simulink library "halout"  (R2021b)
settings: Solver=VariableStepAuto  StartTime=0.0  StopTime=10.0  RelTol=1e-3
undefined symbols (not defined in the file): C_TASK_5MS_S, FALSE, KHAL_CAN1FD1APS3E2E_flg, KHAL_CAN1FD1APS3TxReq_flg, KHAL_CAN1FD1VCU2E2E_flg, KHAL_CAN1FD1VCU2TxReq_flg, KHAL_CAN1FD1VCU3E2E_flg, KHAL_CAN1FD1VCU3TxReq_flg, KHAL_CAN1TxReq_flg, KHAL_CAN1VMCFCM1E2E_flg, KHAL_CAN1VMCFCM1TxReq_flg, KHAL_CAN2TxReq_flg, KHAL_CAN3FD3VCU1toNIDECTxReq_flg, KHAL_CAN3FD3VCU1TxReq_flg, KHAL_CAN3FD3VCU2E2E_flg, KHAL_CAN3FD3VCU2toNIDECE2E_flg, KHAL_CAN3FD3VCU2toNIDECTxReq_flg, KHAL_CAN3FD3VCU2TxReq_flg, KHAL_CAN3TxReq_flg, KHAL_CAN4FD4CE1000E2E_flg, KHAL_CAN4FD4CE1000TxReq_flg, KHAL_CAN4TxReq_flg, KHAL_CAN5TxReq_flg, KHAL_CAN6FD6APS3E2E_flg, KHAL_CAN6FD6APS3TxReq_flg, KHAL_CAN6FD6VCU2E2E_flg, KHAL_CAN6FD6VCU2TxReq_flg, KHAL_CAN6TxReq_flg, ONE_INT, TRUE, ZERO_INT
libraries: FVT_lib x551, simulink x244
(part 22 of 26)

== system halout/HAL_OUT/CAN4/FD4_CE100_0_0x116/Byte_26 ==
  APS_Sta_System : Inport
  CTDLockSW : Inport  Port=2
  CTDUnlockSW : Inport  Port=3
  FDC_VMC_VehPitchAngle_Sta : Inport  Port=4
  BitwiseOR : simulink/Logic and Bit Operations/Bitwise Operator  logicop=OR  UseBitMask=off  NumInputPorts=4  BitMask=bin2dec('11011001')  BitMaskRealWorld=Stored Integer
  SignalPack : FVT_lib/hal/SignalPack  RightShiftCnt=0  BitMask=2^3-1  LeftShiftCnt=3
  SignalPack1 : FVT_lib/hal/SignalPack  RightShiftCnt=0  BitMask=2^1-1  LeftShiftCnt=7
  SignalPack2 : FVT_lib/hal/SignalPack  RightShiftCnt=0  BitMask=2^1-1  LeftShiftCnt=6
  SignalPack3 : FVT_lib/hal/SignalPack  RightShiftCnt=0  BitMask=2^3-1  LeftShiftCnt=0
  UnitConverter{,1..7} (8 alike) : DataTypeConversion  OutDataTypeStr=uint8  RndMeth=Round
  Byte_26 : Outport
  wires:
  BitwiseOR/1 -> Byte_26/1
  UnitConverter/1 -> BitwiseOR/1
  SignalPack/1 -> UnitConverter/1
  UnitConverter1/1 -> SignalPack/1
  APS_Sta_System/1 -> UnitConverter1/1
  UnitConverter2/1 -> BitwiseOR/2
  SignalPack1/1 -> UnitConverter2/1
  UnitConverter3/1 -> SignalPack1/1
  CTDLockSW/1 -> UnitConverter3/1
  UnitConverter4/1 -> BitwiseOR/3
  SignalPack2/1 -> UnitConverter4/1
  UnitConverter5/1 -> SignalPack2/1
  CTDUnlockSW/1 -> UnitConverter5/1
  UnitConverter6/1 -> BitwiseOR/4
  SignalPack3/1 -> UnitConverter6/1
  UnitConverter7/1 -> SignalPack3/1
  FDC_VMC_VehPitchAngle_Sta/1 -> UnitConverter7/1

== system halout/HAL_OUT/CAN4/FD4_CE100_0_0x116/Byte_27 ==
  CtrlDrPwrStbA2 : Inport
  Tailgate_SW : Inport  Port=2
  BitwiseOR : simulink/Logic and Bit Operations/Bitwise Operator  logicop=OR  UseBitMask=off  NumInputPorts=2  BitMask=bin2dec('11011001')  BitMaskRealWorld=Stored Integer
  SignalPack : FVT_lib/hal/SignalPack  RightShiftCnt=0  BitMask=2^1-1  LeftShiftCnt=6
  SignalPack1 : FVT_lib/hal/SignalPack  RightShiftCnt=0  BitMask=2^1-1  LeftShiftCnt=7
  UnitConverter{,1..3} (4 alike) : DataTypeConversion  OutDataTypeStr=uint8  RndMeth=Round
  Byte_27 : Outport
  wires:
  BitwiseOR/1 -> Byte_27/1
  UnitConverter/1 -> BitwiseOR/1
  SignalPack/1 -> UnitConverter/1
  UnitConverter1/1 -> SignalPack/1
  CtrlDrPwrStbA2/1 -> UnitConverter1/1
  UnitConverter2/1 -> BitwiseOR/2
  SignalPack1/1 -> UnitConverter2/1
  UnitConverter3/1 -> SignalPack1/1
  Tailgate_SW/1 -> UnitConverter3/1

== system halout/HAL_OUT/CAN4/FD4_CE100_0_0x116/Byte_3 ==
  H_Beam_ADB : Inport
  PwrSta : Inport  Port=2
  ReBrakeLPReq : Inport  Port=3
  ShiftGearPosn : Inport  Port=4
  BitwiseOR : simulink/Logic and Bit Operations/Bitwise Operator  logicop=OR  UseBitMask=off  NumInputPorts=4  BitMask=bin2dec('11011001')  BitMaskRealWorld=Stored Integer
  SignalPack : FVT_lib/hal/SignalPack  RightShiftCnt=0  BitMask=2^1-1  LeftShiftCnt=0
  SignalPack1 : FVT_lib/hal/SignalPack  RightShiftCnt=0  BitMask=2^3-1  LeftShiftCnt=2
  SignalPack2 : FVT_lib/hal/SignalPack  RightShiftCnt=0  BitMask=2^1-1  LeftShiftCnt=1
  SignalPack3 : FVT_lib/hal/SignalPack  RightShiftCnt=0  BitMask=2^3-1  LeftShiftCnt=5
  UnitConverter{,1..7} (8 alike) : DataTypeConversion  OutDataTypeStr=uint8  RndMeth=Round
  Byte_3 : Outport
  wires:
  BitwiseOR/1 -> Byte_3/1
  UnitConverter/1 -> BitwiseOR/1
  SignalPack/1 -> UnitConverter/1
  UnitConverter1/1 -> SignalPack/1
  H_Beam_ADB/1 -> UnitConverter1/1
  UnitConverter2/1 -> BitwiseOR/2
  SignalPack1/1 -> UnitConverter2/1
  UnitConverter3/1 -> SignalPack1/1
  PwrSta/1 -> UnitConverter3/1
  UnitConverter4/1 -> BitwiseOR/3
  SignalPack2/1 -> UnitConverter4/1
  UnitConverter5/1 -> SignalPack2/1
  ReBrakeLPReq/1 -> UnitConverter5/1
  UnitConverter6/1 -> BitwiseOR/4
  SignalPack3/1 -> UnitConverter6/1
  UnitConverter7/1 -> SignalPack3/1
  ShiftGearPosn/1 -> UnitConverter7/1

== system halout/HAL_OUT/CAN4/FD4_CE100_0_0x116/Byte_4 ==
  DKCTimeSN : Inport
  BitwiseOR : simulink/Logic and Bit Operations/Bitwise Operator  logicop=OR  UseBitMask=off  BitMask=bin2dec('11011001')  BitMaskRealWorld=Stored Integer
  SignalPack : FVT_lib/hal/SignalPack  RightShiftCnt=24  BitMask=2^8-1  LeftShiftCnt=0
  UnitConverter : DataTypeConversion  OutDataTypeStr=uint8  RndMeth=Round
  UnitConverter1 : DataTypeConversion  OutDataTypeStr=uint32  RndMeth=Round
  Byte_4 : Outport
  wires:
  BitwiseOR/1 -> Byte_4/1
  UnitConverter/1 -> BitwiseOR/1
  SignalPack/1 -> UnitConverter/1
  UnitConverter1/1 -> SignalPack/1
  DKCTimeSN/1 -> UnitConverter1/1

== system halout/HAL_OUT/CAN4/FD4_CE100_0_0x116/Byte_5 ==
  DKCTimeSN : Inport
  BitwiseOR : simulink/Logic and Bit Operations/Bitwise Operator  logicop=OR  UseBitMask=off  BitMask=bin2dec('11011001')  BitMaskRealWorld=Stored Integer
  SignalPack : FVT_lib/hal/SignalPack  RightShiftCnt=16  BitMask=2^8-1  LeftShiftCnt=0
  UnitConverter : DataTypeConversion  OutDataTypeStr=uint8  RndMeth=Round
  UnitConverter1 : DataTypeConversion  OutDataTypeStr=uint32  RndMeth=Round
  Byte_5 : Outport
  wires:
  BitwiseOR/1 -> Byte_5/1
  UnitConverter/1 -> BitwiseOR/1
  SignalPack/1 -> UnitConverter/1
  UnitConverter1/1 -> SignalPack/1
  DKCTimeSN/1 -> UnitConverter1/1

== system halout/HAL_OUT/CAN4/FD4_CE100_0_0x116/Byte_6 ==
  DKCTimeSN : Inport
  BitwiseOR : simulink/Logic and Bit Operations/Bitwise Operator  logicop=OR  UseBitMask=off  BitMask=bin2dec('11011001')  BitMaskRealWorld=Stored Integer
  SignalPack : FVT_lib/hal/SignalPack  RightShiftCnt=8  BitMask=2^8-1  LeftShiftCnt=0
  UnitConverter : DataTypeConversion  OutDataTypeStr=uint8  RndMeth=Round
  UnitConverter1 : DataTypeConversion  OutDataTypeStr=uint32  RndMeth=Round
  Byte_6 : Outport
  wires:
  BitwiseOR/1 -> Byte_6/1
  UnitConverter/1 -> BitwiseOR/1
  SignalPack/1 -> UnitConverter/1
  UnitConverter1/1 -> SignalPack/1
  DKCTimeSN/1 -> UnitConverter1/1

== system halout/HAL_OUT/CAN4/FD4_CE100_0_0x116/Byte_7 ==
  DKCTimeSN : Inport
  BitwiseOR : simulink/Logic and Bit Operations/Bitwise Operator  logicop=OR  UseBitMask=off  BitMask=bin2dec('11011001')  BitMaskRealWorld=Stored Integer
  SignalPack : FVT_lib/hal/SignalPack  RightShiftCnt=0  BitMask=2^8-1  LeftShiftCnt=0
  UnitConverter : DataTypeConversion  OutDataTypeStr=uint8  RndMeth=Round
  UnitConverter1 : DataTypeConversion  OutDataTypeStr=uint32  RndMeth=Round
  Byte_7 : Outport
  wires:
  BitwiseOR/1 -> Byte_7/1
  UnitConverter/1 -> BitwiseOR/1
  SignalPack/1 -> UnitConverter/1
  UnitConverter1/1 -> SignalPack/1
  DKCTimeSN/1 -> UnitConverter1/1

== system halout/HAL_OUT/CAN4/FD4_CE100_0_0x116/Byte_8 ==
  TimeSNDKCFbk : Inport
  BitwiseOR : simulink/Logic and Bit Operations/Bitwise Operator  logicop=OR  UseBitMask=off  BitMask=bin2dec('11011001')  BitMaskRealWorld=Stored Integer
  SignalPack : FVT_lib/hal/SignalPack  RightShiftCnt=24  BitMask=2^8-1  LeftShiftCnt=0
  UnitConverter : DataTypeConversion  OutDataTypeStr=uint8  RndMeth=Round
  UnitConverter1 : DataTypeConversion  OutDataTypeStr=uint32  RndMeth=Round
  Byte_8 : Outport
  wires:
  BitwiseOR/1 -> Byte_8/1
  UnitConverter/1 -> BitwiseOR/1
  SignalPack/1 -> UnitConverter/1
  UnitConverter1/1 -> SignalPack/1
  TimeSNDKCFbk/1 -> UnitConverter1/1

== system halout/HAL_OUT/CAN4/FD4_CE100_0_0x116/Byte_9 ==
  TimeSNDKCFbk : Inport
  BitwiseOR : simulink/Logic and Bit Operations/Bitwise Operator  logicop=OR  UseBitMask=off  BitMask=bin2dec('11011001')  BitMaskRealWorld=Stored Integer
  SignalPack : FVT_lib/hal/SignalPack  RightShiftCnt=16  BitMask=2^8-1  LeftShiftCnt=0
  UnitConverter : DataTypeConversion  OutDataTypeStr=uint8  RndMeth=Round
  UnitConverter1 : DataTypeConversion  OutDataTypeStr=uint32  RndMeth=Round
  Byte_9 : Outport
  wires:
  BitwiseOR/1 -> Byte_9/1
  UnitConverter/1 -> BitwiseOR/1
  SignalPack/1 -> UnitConverter/1
  UnitConverter1/1 -> SignalPack/1
  TimeSNDKCFbk/1 -> UnitConverter1/1

== system halout/HAL_OUT/CAN4/FD4_CE100_0_0x116/CCCrlSta ==
  CCCrlSta : Inport
  Data Type Conversion : DataTypeConversion  OutDataTypeStr=uint8  RndMeth=Round
  CAN4_CC_Crl_Sta : Outport
  wires:
  Data Type Conversion/1 -> CAN4_CC_Crl_Sta/1
  CCCrlSta/1 -> Data Type Conversion/1

== system halout/HAL_OUT/CAN4/FD4_CE100_0_0x116/CRC8_IfAction_Tx ==
  CAN_E2E_flg : Inport
  DataID1 : Inport  Port=2
  DataID2 : Inport  Port=3
  RawData : Inport  Port=4
  Data Type Conversion : DataTypeConversion  OutDataTypeStr=uint8
  If : If
  If Action Subsystem : Subsystem  TreatAsAtomicUnit=on
  If Action Subsystem1 : Subsystem  TreatAsAtomicUnit=on
  Merge : Merge
  CRC8 : Outport
  wires:
  If/2 -> If Action Subsystem/Action
  If/1 -> If Action Subsystem1/Action
  CAN_E2E_flg/1 -> [CAN_E2E_flg]
  DataID1/1 -> [DataID1]
  DataID2/1 -> [DataID2]
  RawData/1 -> [RawData]
  [CAN_E2E_flg] -> Data Type Conversion/1
  [DataID1] -> If Action Subsystem1/1(CAN_E2E_ID1)
  [DataID2] -> If Action Subsystem1/2(CAN_E2E_ID2)
  [RawData] -> If Action Subsystem1/3(Byte1)
  [RawData] -> If Action Subsystem/1(Byte1)
  If Action Subsystem1/1(CRC8_E2EResult) -> Merge/1
  If Action Subsystem/1(CRC8_Result) -> Merge/2
  Merge/1 -> CRC8/1
  Data Type Conversion/1 -> If/1

== system halout/HAL_OUT/CAN4/FD4_CE100_0_0x116/CSVCU1CAN4 ==
  CSVCU1CAN4 : Inport
  Data Type Conversion : DataTypeConversion  OutDataTypeStr=uint8  RndMeth=Round
  CAN4_CS_VCU1_CAN4 : Outport
  wires:
  Data Type Conversion/1 -> CAN4_CS_VCU1_CAN4/1
  CSVCU1CAN4/1 -> Data Type Conversion/1

== system halout/HAL_OUT/CAN4/FD4_CE100_0_0x116/CTDCtrl ==
  CTDCtrl : Inport
  Data Type Conversion : DataTypeConversion  OutDataTypeStr=uint8  RndMeth=Round
  CAN4_CTDCtrl : Outport
  wires:
  Data Type Conversion/1 -> CAN4_CTDCtrl/1
  CTDCtrl/1 -> Data Type Conversion/1

== system halout/HAL_OUT/CAN4/FD4_CE100_0_0x116/CTDLockSW ==
  CTDLockSW : Inport
  Data Type Conversion : DataTypeConversion  OutDataTypeStr=uint8  RndMeth=Round
  CAN4_CTDLockSW : Outport
  wires:
  Data Type Conversion/1 -> CAN4_CTDLockSW/1
  CTDLockSW/1 -> Data Type Conversion/1

== system halout/HAL_OUT/CAN4/FD4_CE100_0_0x116/CTDUnlockSW ==
  CTDUnlockSW : Inport
  Data Type Conversion : DataTypeConversion  OutDataTypeStr=uint8  RndMeth=Round
  CAN4_CTDUnlockSW : Outport
  wires:
  Data Type Conversion/1 -> CAN4_CTDUnlockSW/1
  CTDUnlockSW/1 -> Data Type Conversion/1

== system halout/HAL_OUT/CAN4/FD4_CE100_0_0x116/CrashDetd ==
  CrashDetd : Inport
  Data Type Conversion : DataTypeConversion  OutDataTypeStr=uint8  RndMeth=Round
  CAN4_CrashDetd : Outport
  wires:
  Data Type Conversion/1 -> CAN4_CrashDetd/1
  CrashDetd/1 -> Data Type Conversion/1

== system halout/HAL_OUT/CAN4/FD4_CE100_0_0x116/CtrlDrPwrStbA2 ==
  CtrlDrPwrStbA2 : Inport
  Data Type Conversion : DataTypeConversion  OutDataTypeStr=uint8  RndMeth=Round
  CAN4_CtrlDrPwrStbA2 : Outport
  wires:
  Data Type Conversion/1 -> CAN4_CtrlDrPwrStbA2/1
  CtrlDrPwrStbA2/1 -> Data Type Conversion/1

== system halout/HAL_OUT/CAN4/FD4_CE100_0_0x116/CtrlFrBMSCCUCIR ==
  CtrlFrBMSCCUCIR : Inport
  Data Type Conversion : DataTypeConversion  OutDataTypeStr=uint8  RndMeth=Round
  CAN4_CtrlFrBMSCCUCIR : Outport
  wires:
  Data Type Conversion/1 -> CAN4_CtrlFrBMSCCUCIR/1
  CtrlFrBMSCCUCIR/1 -> Data Type Conversion/1

== system halout/HAL_OUT/CAN4/FD4_CE100_0_0x116/CtrlFrEDUINVERTER ==
  CtrlFrEDUINVERTER : Inport
  Data Type Conversion : DataTypeConversion  OutDataTypeStr=uint8  RndMeth=Round
  CAN4_CtrlFrEDUINVERTER : Outport
  wires:
  Data Type Conversion/1 -> CAN4_CtrlFrEDUINVERTER/1
  CtrlFrEDUINVERTER/1 -> Data Type Conversion/1

== system halout/HAL_OUT/CAN4/FD4_CE100_0_0x116/CtrlFrIRC1 ==
  CtrlFrIRC1 : Inport
  Data Type Conversion : DataTypeConversion  OutDataTypeStr=uint8  RndMeth=Round
  CAN4_CtrlFrIRC1 : Outport
  wires:
  Data Type Conversion/1 -> CAN4_CtrlFrIRC1/1
  CtrlFrIRC1/1 -> Data Type Conversion/1

== system halout/HAL_OUT/CAN4/FD4_CE100_0_0x116/CtrlFrPwrStbA1P ==
  CtrlFrPwrStbA1P : Inport
  Data Type Conversion : DataTypeConversion  OutDataTypeStr=uint8  RndMeth=Round
  CAN4_CtrlFrPwrStbA1P : Outport
  wires:
  Data Type Conversion/1 -> CAN4_CtrlFrPwrStbA1P/1
  CtrlFrPwrStbA1P/1 -> Data Type Conversion/1

== system halout/HAL_OUT/CAN4/FD4_CE100_0_0x116/DKCAuthSta ==
  DKCAuthSta : Inport
  Data Type Conversion : DataTypeConversion  OutDataTypeStr=uint8  RndMeth=Round
  CAN4_DKCAuthSta : Outport
  wires:
  Data Type Conversion/1 -> CAN4_DKCAuthSta/1
  DKCAuthSta/1 -> Data Type Conversion/1

== system halout/HAL_OUT/CAN4/FD4_CE100_0_0x116/DKCTimeSN ==
  DKCTimeSN : Inport
  Data Type Conversion : DataTypeConversion  OutDataTypeStr=uint32  RndMeth=Round
  CAN4_DKCTimeSN : Outport
  wires:
  Data Type Conversion/1 -> CAN4_DKCTimeSN/1
  DKCTimeSN/1 -> Data Type Conversion/1

== system halout/HAL_OUT/CAN4/FD4_CE100_0_0x116/Dimmer ==
  Dimmer : Inport
  Data Type Conversion : DataTypeConversion  OutDataTypeStr=uint8  RndMeth=Round
  CAN4_Dimmer : Outport
  wires:
  Data Type Conversion/1 -> CAN4_Dimmer/1
  Dimmer/1 -> Data Type Conversion/1

== system halout/HAL_OUT/CAN4/FD4_CE100_0_0x116/DimmerEN ==
  DimmerEN : Inport
  Data Type Conversion : DataTypeConversion  OutDataTypeStr=uint8  RndMeth=Round
  CAN4_DimmerEN : Outport
  wires:
  Data Type Conversion/1 -> CAN4_DimmerEN/1
  DimmerEN/1 -> Data Type Conversion/1

== system halout/HAL_OUT/CAN4/FD4_CE100_0_0x116/DoorLockIND ==
  DoorLockIND : Inport
  Data Type Conversion : DataTypeConversion  OutDataTypeStr=uint8  RndMeth=Round
  CAN4_DoorLockIND : Outport
  wires:
  Data Type Conversion/1 -> CAN4_DoorLockIND/1
  DoorLockIND/1 -> Data Type Conversion/1

== system halout/HAL_OUT/CAN4/FD4_CE100_0_0x116/DrDoorSW ==
  DrDoorSW : Inport
  Data Type Conversion : DataTypeConversion  OutDataTypeStr=uint8  RndMeth=Round
  CAN4_DrDoorSW : Outport
  wires:
  Data Type Conversion/1 -> CAN4_DrDoorSW/1
  DrDoorSW/1 -> Data Type Conversion/1

== system halout/HAL_OUT/CAN4/FD4_CE100_0_0x116/DrSeatSta ==
  DrSeatSta : Inport
  Data Type Conversion : DataTypeConversion  OutDataTypeStr=uint8  RndMeth=Round
  CAN4_Dr_SeatSta : Outport
  wires:
  Data Type Conversion/1 -> CAN4_Dr_SeatSta/1
  DrSeatSta/1 -> Data Type Conversion/1

== system halout/HAL_OUT/CAN4/FD4_CE100_0_0x116/EquivAccPedalSWSta ==
  EquivAccPedalSWSta : Inport
  Data Type Conversion : DataTypeConversion  OutDataTypeStr=uint8  RndMeth=Round
  CAN4_EquivAccPedalSWSta : Outport
  wires:
  Data Type Conversion/1 -> CAN4_EquivAccPedalSWSta/1
  EquivAccPedalSWSta/1 -> Data Type Conversion/1

== system halout/HAL_OUT/CAN4/FD4_CE100_0_0x116/FDCVMCVehPitchAngleSta ==
  FDCVMCVehPitchAngleSta : Inport
  Data Type Conversion : DataTypeConversion  OutDataTypeStr=uint8  RndMeth=Round
  CAN4_FDC_VMC_VehPitchAngle_Sta : Outport
  wires:
  Data Type Conversion/1 -> CAN4_FDC_VMC_VehPitchAngle_Sta/1
  FDCVMCVehPitchAngleSta/1 -> Data Type Conversion/1

== system halout/HAL_OUT/CAN4/FD4_CE100_0_0x116/FDDKCVehDataErr ==
  FDDKCVehDataErr : Inport
  Data Type Conversion : DataTypeConversion  OutDataTypeStr=uint8  RndMeth=Round
  CAN4_FD_DKC_VehData_Err : Outport
  wires:
  Data Type Conversion/1 -> CAN4_FD_DKC_VehData_Err/1
  FDDKCVehDataErr/1 -> Data Type Conversion/1

== system halout/HAL_OUT/CAN4/FD4_CE100_0_0x116/FDDKCVehDataSta ==
  FDDKCVehDataSta : Inport
  Data Type Conversion : DataTypeConversion  OutDataTypeStr=uint8  RndMeth=Round
  CAN4_FD_DKC_VehData_Sta : Outport
  wires:
  Data Type Conversion/1 -> CAN4_FD_DKC_VehData_Sta/1
  FDDKCVehDataSta/1 -> Data Type Conversion/1

== system halout/HAL_OUT/CAN4/FD4_CE100_0_0x116/FDTBOXDTCDataErr ==
  FDTBOXDTCDataErr : Inport
  Data Type Conversion : DataTypeConversion  OutDataTypeStr=uint8  RndMeth=Round
  CAN4_FD_TBOX_DTCData_Err : Outport
  wires:
  Data Type Conversion/1 -> CAN4_FD_TBOX_DTCData_Err/1
  FDTBOXDTCDataErr/1 -> Data Type Conversion/1

== system halout/HAL_OUT/CAN4/FD4_CE100_0_0x116/FDTBOXDTCDataSta ==
  FDTBOXDTCDataSta : Inport
  Data Type Conversion : DataTypeConversion  OutDataTypeStr=uint8  RndMeth=Round
  CAN4_FD_TBOX_DTCData_Sta : Outport
  wires:
  Data Type Conversion/1 -> CAN4_FD_TBOX_DTCData_Sta/1
  FDTBOXDTCDataSta/1 -> Data Type Conversion/1

== system halout/HAL_OUT/CAN4/FD4_CE100_0_0x116/FDTBOXVehDataErr ==
  FDTBOXVehDataErr : Inport
  Data Type Conversion : DataTypeConversion  OutDataTypeStr=uint8  RndMeth=Round
  CAN4_FD_TBOX_VehData_Err : Outport
  wires:
  Data Type Conversion/1 -> CAN4_FD_TBOX_VehData_Err/1
  FDTBOXVehDataErr/1 -> Data Type Conversion/1

== system halout/HAL_OUT/CAN4/FD4_CE100_0_0x116/FDTBOXVehDataSta ==
  FDTBOXVehDataSta : Inport
  Data Type Conversion : DataTypeConversion  OutDataTypeStr=uint8  RndMeth=Round
  CAN4_FD_TBOX_VehData_Sta : Outport
  wires:
  Data Type Conversion/1 -> CAN4_FD_TBOX_VehData_Sta/1
  FDTBOXVehDataSta/1 -> Data Type Conversion/1

== system halout/HAL_OUT/CAN4/FD4_CE100_0_0x116/FrChargingDoorCtrl ==
  FrChargingDoorCtrl : Inport
  Data Type Conversion : DataTypeConversion  OutDataTypeStr=uint8  RndMeth=Round
  CAN4_Fr_ChargingDoorCtrl : Outport
  wires:
  Data Type Conversion/1 -> CAN4_Fr_ChargingDoorCtrl/1
  FrChargingDoorCtrl/1 -> Data Type Conversion/1

== system halout/HAL_OUT/CAN4/FD4_CE100_0_0x116/FrFogLamp ==
  FrFogLamp : Inport
  Data Type Conversion : DataTypeConversion  OutDataTypeStr=uint8  RndMeth=Round
  CAN4_Fr_FogLamp : Outport
  wires:
  Data Type Conversion/1 -> CAN4_Fr_FogLamp/1
  FrFogLamp/1 -> Data Type Conversion/1

== system halout/HAL_OUT/CAN4/FD4_CE100_0_0x116/FrWiperH ==
  FrWiperH : Inport
  Data Type Conversion : DataTypeConversion  OutDataTypeStr=uint8  RndMeth=Round
  CAN4_Fr_Wiper_H : Outport
  wires:
  Data Type Conversion/1 -> CAN4_Fr_Wiper_H/1
  FrWiperH/1 -> Data Type Conversion/1

== system halout/HAL_OUT/CAN4/FD4_CE100_0_0x116/FrWiperL ==
  FrWiperL : Inport
  Data Type Conversion : DataTypeConversion  OutDataTypeStr=uint8  RndMeth=Round
  CAN4_Fr_Wiper_L : Outport
  wires:
  Data Type Conversion/1 -> CAN4_Fr_Wiper_L/1
  FrWiperL/1 -> Data Type Conversion/1

== system halout/HAL_OUT/CAN4/FD4_CE100_0_0x116/HBeam ==
  HBeam : Inport
  Data Type Conversion : DataTypeConversion  OutDataTypeStr=uint8  RndMeth=Round
  CAN4_H_Beam : Outport
  wires:
  Data Type Conversion/1 -> CAN4_H_Beam/1
  HBeam/1 -> Data Type Conversion/1

== system halout/HAL_OUT/CAN4/FD4_CE100_0_0x116/HBeamADB ==
  HBeamADB : Inport
  Data Type Conversion : DataTypeConversion  OutDataTypeStr=uint8  RndMeth=Round
  CAN4_H_Beam_ADB : Outport
  wires:
  Data Type Conversion/1 -> CAN4_H_Beam_ADB/1
  HBeamADB/1 -> Data Type Conversion/1

== system halout/HAL_OUT/CAN4/FD4_CE100_0_0x116/HWResetSta ==
  HWResetSta : Inport
  Data Type Conversion : DataTypeConversion  OutDataTypeStr=uint8  RndMeth=Round
  CAN4_HWResetSta : Outport
  wires:
  Data Type Conversion/1 -> CAN4_HWResetSta/1
  HWResetSta/1 -> Data Type Conversion/1

== system halout/HAL_OUT/CAN4/FD4_CE100_0_0x116/HazardSW ==
  HazardSW : Inport
  Data Type Conversion : DataTypeConversion  OutDataTypeStr=uint8  RndMeth=Round
  CAN4_HazardSW : Outport
  wires:
  Data Type Conversion/1 -> CAN4_HazardSW/1
  HazardSW/1 -> Data Type Conversion/1

== system halout/HAL_OUT/CAN4/FD4_CE100_0_0x116/HoodSW ==
  HoodSW : Inport
  Data Type Conversion : DataTypeConversion  OutDataTypeStr=uint8  RndMeth=Round
  CAN4_HoodSW : Outport
  wires:
  Data Type Conversion/1 -> CAN4_HoodSW/1
  HoodSW/1 -> Data Type Conversion/1

== system halout/HAL_OUT/CAN4/FD4_CE100_0_0x116/HornCtrl ==
  HornCtrl : Inport
  Data Type Conversion : DataTypeConversion  OutDataTypeStr=uint8  RndMeth=Round
  CAN4_HornCtrl : Outport
  wires:
  Data Type Conversion/1 -> CAN4_HornCtrl/1
  HornCtrl/1 -> Data Type Conversion/1

== system halout/HAL_OUT/CAN4/FD4_CE100_0_0x116/LAPMWdwEnable ==
  LAPMWdwEnable : Inport
  Data Type Conversion : DataTypeConversion  OutDataTypeStr=uint8  RndMeth=Round
  CAN4_L_APM_WdwEnable : Outport
  wires:
  Data Type Conversion/1 -> CAN4_L_APM_WdwEnable/1
  LAPMWdwEnable/1 -> Data Type Conversion/1

== system halout/HAL_OUT/CAN4/FD4_CE100_0_0x116/LBSD ==
  LBSD : Inport
  Data Type Conversion : DataTypeConversion  OutDataTypeStr=uint8  RndMeth=Round
  CAN4_LBSD : Outport
  wires:
  Data Type Conversion/1 -> CAN4_LBSD/1
  LBSD/1 -> Data Type Conversion/1

== system halout/HAL_OUT/CAN4/FD4_CE100_0_0x116/LBeam ==
  LBeam : Inport
  Data Type Conversion : DataTypeConversion  OutDataTypeStr=uint8  RndMeth=Round
  CAN4_L_Beam : Outport
  wires:
  Data Type Conversion/1 -> CAN4_L_Beam/1
  LBeam/1 -> Data Type Conversion/1

== system halout/HAL_OUT/CAN4/FD4_CE100_0_0x116/LDRL ==
  LDRL : Inport
  Data Type Conversion : DataTypeConversion  OutDataTypeStr=uint8  RndMeth=Round
  CAN4_LDRL : Outport
  wires:
  Data Type Conversion/1 -> CAN4_LDRL/1
  LDRL/1 -> Data Type Conversion/1

== system halout/HAL_OUT/CAN4/FD4_CE100_0_0x116/LTurnLP ==
  LTurnLP : Inport
  Data Type Conversion : DataTypeConversion  OutDataTypeStr=uint8  RndMeth=Round
  CAN4_LTurnLP : Outport
  wires:
  Data Type Conversion/1 -> CAN4_LTurnLP/1
  LTurnLP/1 -> Data Type Conversion/1

== system halout/HAL_OUT/CAN4/FD4_CE100_0_0x116/LampPwr ==
  LampPwr : Inport
  Data Type Conversion : DataTypeConversion  OutDataTypeStr=uint8  RndMeth=Round
  CAN4_LampPwr : Outport
  wires:
  Data Type Conversion/1 -> CAN4_LampPwr/1
  LampPwr/1 -> Data Type Conversion/1

== system halout/HAL_OUT/CAN4/FD4_CE100_0_0x116/LockSetting ==
  LockSetting : Inport
  Data Type Conversion : DataTypeConversion  OutDataTypeStr=uint8  RndMeth=Round
  CAN4_LockSetting : Outport
  wires:
  Data Type Conversion/1 -> CAN4_LockSetting/1
  LockSetting/1 -> Data Type Conversion/1

== system halout/HAL_OUT/CAN4/FD4_CE100_0_0x116/MSACrlSta ==
  MSACrlSta : Inport
  Data Type Conversion : DataTypeConversion  OutDataTypeStr=uint8  RndMeth=Round
  CAN4_MSA_Crl_Sta : Outport
  wires:
  Data Type Conversion/1 -> CAN4_MSA_Crl_Sta/1
  MSACrlSta/1 -> Data Type Conversion/1

== system halout/HAL_OUT/CAN4/FD4_CE100_0_0x116/MirrorCtrl ==
  MirrorCtrl : Inport
  Data Type Conversion : DataTypeConversion  OutDataTypeStr=uint8  RndMeth=Round
  CAN4_MirrorCtrl : Outport
  wires:
  Data Type Conversion/1 -> CAN4_MirrorCtrl/1
  MirrorCtrl/1 -> Data Type Conversion/1

== system halout/HAL_OUT/CAN4/FD4_CE100_0_0x116/MirrorDefog ==
  MirrorDefog : Inport
  Data Type Conversion : DataTypeConversion  OutDataTypeStr=uint8  RndMeth=Round
  CAN4_MirrorDefog : Outport
  wires:
  Data Type Conversion/1 -> CAN4_MirrorDefog/1
  MirrorDefog/1 -> Data Type Conversion/1

== system halout/HAL_OUT/CAN4/FD4_CE100_0_0x116/PosLamp ==
  PosLamp : Inport
  Data Type Conversion : DataTypeConversion  OutDataTypeStr=uint8  RndMeth=Round
  CAN4_PosLamp : Outport
  wires:
  Data Type Conversion/1 -> CAN4_PosLamp/1
  PosLamp/1 -> Data Type Conversion/1

== system halout/HAL_OUT/CAN4/FD4_CE100_0_0x116/PsDoorSW ==
  PsDoorSW : Inport
  Data Type Conversion : DataTypeConversion  OutDataTypeStr=uint8  RndMeth=Round
  CAN4_PsDoorSW : Outport
  wires:
  Data Type Conversion/1 -> CAN4_PsDoorSW/1
  PsDoorSW/1 -> Data Type Conversion/1

== system halout/HAL_OUT/CAN4/FD4_CE100_0_0x116/PwrSta ==
  PwrSta : Inport
  Data Type Conversion : DataTypeConversion  OutDataTypeStr=uint8  RndMeth=Round
  CAN4_PwrSta : Outport
  wires:
  Data Type Conversion/1 -> CAN4_PwrSta/1
  PwrSta/1 -> Data Type Conversion/1

== system halout/HAL_OUT/CAN4/FD4_CE100_0_0x116/RBSD ==
  RBSD : Inport
  Data Type Conversion : DataTypeConversion  OutDataTypeStr=uint8  RndMeth=Round
  CAN4_RBSD : Outport
  wires:
  Data Type Conversion/1 -> CAN4_RBSD/1
  RBSD/1 -> Data Type Conversion/1

== system halout/HAL_OUT/CAN4/FD4_CE100_0_0x116/RCVCU1CAN4 ==
  RCVCU1CAN4 : Inport
  Data Type Conversion : DataTypeConversion  OutDataTypeStr=uint8  RndMeth=Round
  CAN4_RC_VCU1_CAN4 : Outport
  wires:
  Data Type Conversion/1 -> CAN4_RC_VCU1_CAN4/1
  RCVCU1CAN4/1 -> Data Type Conversion/1

== system halout/HAL_OUT/CAN4/FD4_CE100_0_0x116/RDRL ==
  RDRL : Inport
  Data Type Conversion : DataTypeConversion  OutDataTypeStr=uint8  RndMeth=Round
  CAN4_RDRL : Outport
  wires:
  Data Type Conversion/1 -> CAN4_RDRL/1
  RDRL/1 -> Data Type Conversion/1

== system halout/HAL_OUT/CAN4/FD4_CE100_0_0x116/RLDoorSW ==
  RLDoorSW : Inport
  Data Type Conversion : DataTypeConversion  OutDataTypeStr=uint8  RndMeth=Round
  CAN4_RLDoorSW : Outport
  wires:
  Data Type Conversion/1 -> CAN4_RLDoorSW/1
  RLDoorSW/1 -> Data Type Conversion/1

== system halout/HAL_OUT/CAN4/FD4_CE100_0_0x116/RRDoorSW ==
  RRDoorSW : Inport
  Data Type Conversion : DataTypeConversion  OutDataTypeStr=uint8  RndMeth=Round
  CAN4_RRDoorSW : Outport
  wires:
  Data Type Conversion/1 -> CAN4_RRDoorSW/1
  RRDoorSW/1 -> Data Type Conversion/1

== system halout/HAL_OUT/CAN4/FD4_CE100_0_0x116/RTurnLP ==
  RTurnLP : Inport
  Data Type Conversion : DataTypeConversion  OutDataTypeStr=uint8  RndMeth=Round
  CAN4_RTurnLP : Outport
  wires:
  Data Type Conversion/1 -> CAN4_RTurnLP/1
  RTurnLP/1 -> Data Type Conversion/1

== system halout/HAL_OUT/CAN4/FD4_CE100_0_0x116/ReBrakeLPReq ==
  ReBrakeLPReq : Inport
  Data Type Conversion : DataTypeConversion  OutDataTypeStr=uint8  RndMeth=Round
  CAN4_ReBrakeLPReq : Outport
  wires:
  Data Type Conversion/1 -> CAN4_ReBrakeLPReq/1
  ReBrakeLPReq/1 -> Data Type Conversion/1

== system halout/HAL_OUT/CAN4/FD4_CE100_0_0x116/ReverseLamp ==
  ReverseLamp : Inport
  Data Type Conversion : DataTypeConversion  OutDataTypeStr=uint8  RndMeth=Round
  CAN4_ReverseLamp : Outport
  wires:
  Data Type Conversion/1 -> CAN4_ReverseLamp/1
  ReverseLamp/1 -> Data Type Conversion/1

== system halout/HAL_OUT/CAN4/FD4_CE100_0_0x116/RoomLampH ==
  RoomLampH : Inport
  Data Type Conversion : DataTypeConversion  OutDataTypeStr=uint8  RndMeth=Round
  CAN4_RoomLampH : Outport
  wires:
  Data Type Conversion/1 -> CAN4_RoomLampH/1
  RoomLampH/1 -> Data Type Conversion/1

== system halout/HAL_OUT/CAN4/FD4_CE100_0_0x116/RoomLampL ==
  RoomLampL : Inport
  Data Type Conversion : DataTypeConversion  OutDataTypeStr=uint8  RndMeth=Round
  CAN4_RoomLampL : Outport
  wires:
  Data Type Conversion/1 -> CAN4_RoomLampL/1
  RoomLampL/1 -> Data Type Conversion/1

== system halout/HAL_OUT/CAN4/FD4_CE100_0_0x116/RrChargingDoorCtrl ==
  RrChargingDoorCtrl : Inport
  Data Type Conversion : DataTypeConversion  OutDataTypeStr=uint8  RndMeth=Round
  CAN4_Rr_ChargingDoorCtrl : Outport
  wires:
  Data Type Conversion/1 -> CAN4_Rr_ChargingDoorCtrl/1
  RrChargingDoorCtrl/1 -> Data Type Conversion/1

== system halout/HAL_OUT/CAN4/FD4_CE100_0_0x116/RrDefog ==
  RrDefog : Inport
  Data Type Conversion : DataTypeConversion  OutDataTypeStr=uint8  RndMeth=Round
  CAN4_Rr_Defog : Outport
  wires:
  Data Type Conversion/1 -> CAN4_Rr_Defog/1
  RrDefog/1 -> Data Type Conversion/1

== system halout/HAL_OUT/CAN4/FD4_CE100_0_0x116/RrFogLamp ==
  RrFogLamp : Inport
  Data Type Conversion : DataTypeConversion  OutDataTypeStr=uint8  RndMeth=Round
  CAN4_Rr_FogLamp : Outport
  wires:
  Data Type Conversion/1 -> CAN4_Rr_FogLamp/1
  RrFogLamp/1 -> Data Type Conversion/1

== system halout/HAL_OUT/CAN4/FD4_CE100_0_0x116/RrWiper ==
  RrWiper : Inport
  Data Type Conversion : DataTypeConversion  OutDataTypeStr=uint8  RndMeth=Round
  CAN4_Rr_Wiper : Outport
  wires:
  Data Type Conversion/1 -> CAN4_Rr_Wiper/1
  RrWiper/1 -> Data Type Conversion/1

== system halout/HAL_OUT/CAN4/FD4_CE100_0_0x116/ShiftGearPosn ==
  ShiftGearPosn : Inport
  Data Type Conversion : DataTypeConversion  OutDataTypeStr=uint8  RndMeth=Round
  CAN4_ShiftGearPosn : Outport
  wires:
  Data Type Conversion/1 -> CAN4_ShiftGearPosn/1
  ShiftGearPosn/1 -> Data Type Conversion/1

== system halout/HAL_OUT/CAN4/FD4_CE100_0_0x116/TailgateHDSW ==
  TailgateHDSW : Inport
  Data Type Conversion : DataTypeConversion  OutDataTypeStr=uint8  RndMeth=Round
  CAN4_TailgateHDSW : Outport
  wires:
  Data Type Conversion/1 -> CAN4_TailgateHDSW/1
  TailgateHDSW/1 -> Data Type Conversion/1

== system halout/HAL_OUT/CAN4/FD4_CE100_0_0x116/TailgateRemote ==
  TailgateRemote : Inport
  Data Type Conversion : DataTypeConversion  OutDataTypeStr=uint8  RndMeth=Round
  CAN4_TailgateRemote : Outport
  wires:
  Data Type Conversion/1 -> CAN4_TailgateRemote/1
  TailgateRemote/1 -> Data Type Conversion/1

== system halout/HAL_OUT/CAN4/FD4_CE100_0_0x116/TailgateSW ==
  TailgateSW : Inport
  Data Type Conversion : DataTypeConversion  OutDataTypeStr=uint8  RndMeth=Round
  CAN4_Tailgate_SW : Outport
  wires:
  Data Type Conversion/1 -> CAN4_Tailgate_SW/1
  TailgateSW/1 -> Data Type Conversion/1

== system halout/HAL_OUT/CAN4/FD4_CE100_0_0x116/TimeSNDKCFbk ==
  TimeSNDKCFbk : Inport
  Data Type Conversion : DataTypeConversion  OutDataTypeStr=uint32  RndMeth=Round
  CAN4_TimeSNDKCFbk : Outport
  wires:
  Data Type Conversion/1 -> CAN4_TimeSNDKCFbk/1
  TimeSNDKCFbk/1 -> Data Type Conversion/1

== system halout/HAL_OUT/CAN4/FD4_CE100_0_0x116/TrunkRel ==
  TrunkRel : Inport
  Data Type Conversion : DataTypeConversion  OutDataTypeStr=uint8  RndMeth=Round
  CAN4_TrunkRel : Outport
  wires:
  Data Type Conversion/1 -> CAN4_TrunkRel/1
  TrunkRel/1 -> Data Type Conversion/1

== system halout/HAL_OUT/CAN4/FD4_CE100_0_0x116/WasherCtrl ==
  WasherCtrl : Inport
  Data Type Conversion : DataTypeConversion  OutDataTypeStr=uint8  RndMeth=Round
  CAN4_WasherCtrl : Outport
  wires:
  Data Type Conversion/1 -> CAN4_WasherCtrl/1
  WasherCtrl/1 -> Data Type Conversion/1

== system halout/HAL_OUT/CAN4/FD4_CE100_0_0x116/WiperFixMode ==
  WiperFixMode : Inport
  Data Type Conversion : DataTypeConversion  OutDataTypeStr=uint8  RndMeth=Round
  CAN4_WiperFixMode : Outport
  wires:
  Data Type Conversion/1 -> CAN4_WiperFixMode/1
  WiperFixMode/1 -> Data Type Conversion/1

== system halout/HAL_OUT/CAN4/FD4_CE100_1_0x182/ACSubMode ==
  ACSubMode : Inport
  Data Type Conversion : DataTypeConversion  OutDataTypeStr=uint8  RndMeth=Round
  CAN4_ACSubMode : Outport
  wires:
  Data Type Conversion/1 -> CAN4_ACSubMode/1
  ACSubMode/1 -> Data Type Conversion/1

== system halout/HAL_OUT/CAN4/FD4_CE100_1_0x182/APTCActFrRiPwr ==
  APTCActFrRiPwr : Inport
  Data Type Conversion : DataTypeConversion  OutDataTypeStr=uint8  RndMeth=Round
  convert_out : FVT_lib/hal/convert_out  gain=25  offset=0
  CAN4_APTC_ActFrRiPwr : Outport
  wires:
  Data Type Conversion/1 -> CAN4_APTC_ActFrRiPwr/1
  convert_out/1 -> Data Type Conversion/1
  APTCActFrRiPwr/1 -> convert_out/1

== system halout/HAL_OUT/CAN4/FD4_CE100_1_0x182/BatLoopActWtFlw ==
  BatLoopActWtFlw : Inport
  Data Type Conversion : DataTypeConversion  OutDataTypeStr=uint8  RndMeth=Round
  convert_out : FVT_lib/hal/convert_out  gain=0.1  offset=-5
  CAN4_BatLoopActWtFlw : Outport
  wires:
  Data Type Conversion/1 -> CAN4_BatLoopActWtFlw/1
  convert_out/1 -> Data Type Conversion/1
  BatLoopActWtFlw/1 -> convert_out/1

== system halout/HAL_OUT/CAN4/FD4_CE100_1_0x182/BatteryMode ==
  BatteryMode : Inport
  Data Type Conversion : DataTypeConversion  OutDataTypeStr=uint8  RndMeth=Round
  CAN4_BatteryMode : Outport
  wires:
  Data Type Conversion/1 -> CAN4_BatteryMode/1
  BatteryMode/1 -> Data Type Conversion/1

== system halout/HAL_OUT/CAN4/FD4_CE100_1_0x182/CCUACLampSts ==
  CCUACLampSts : Inport
  Data Type Conversion : DataTypeConversion  OutDataTypeStr=uint8  RndMeth=Round
  CAN4_CCU_ACLampSts : Outport
  wires:
  Data Type Conversion/1 -> CAN4_CCU_ACLampSts/1
  CCUACLampSts/1 -> Data Type Conversion/1

== system halout/HAL_OUT/CAN4/FD4_CE100_1_0x182/CCUACMaxLampSts ==
  CCUACMaxLampSts : Inport
  Data Type Conversion : DataTypeConversion  OutDataTypeStr=uint8  RndMeth=Round
  CAN4_CCU_ACMaxLampSts : Outport
  wires:
  Data Type Conversion/1 -> CAN4_CCU_ACMaxLampSts/1
  CCUACMaxLampSts/1 -> Data Type Conversion/1

== system halout/HAL_OUT/CAN4/FD4_CE100_1_0x182/CCUAutoLampSts ==
  CCUAutoLampSts : Inport
  Data Type Conversion : DataTypeConversion  OutDataTypeStr=uint8  RndMeth=Round
  CAN4_CCU_AutoLampSts : Outport
  wires:
  Data Type Conversion/1 -> CAN4_CCU_AutoLampSts/1
  CCUAutoLampSts/1 -> Data Type Conversion/1

== system halout/HAL_OUT/CAN4/FD4_CE100_1_0x182/CCUAutoMidLampSts ==
  CCUAutoMidLampSts : Inport
  Data Type Conversion : DataTypeConversion  OutDataTypeStr=uint8  RndMeth=Round
  CAN4_CCU_AutoMidLampSts : Outport
  wires:
  Data Type Conversion/1 -> CAN4_CCU_AutoMidLampSts/1
  CCUAutoMidLampSts/1 -> Data Type Conversion/1

== system halout/HAL_OUT/CAN4/FD4_CE100_1_0x182/CCUCbnPreACWkSts ==
  CCUCbnPreACWkSts : Inport
  Data Type Conversion : DataTypeConversion  OutDataTypeStr=uint8  RndMeth=Round
  CAN4_CCU_CbnPreACWkSts : Outport
  wires:
  Data Type Conversion/1 -> CAN4_CCU_CbnPreACWkSts/1
  CCUCbnPreACWkSts/1 -> Data Type Conversion/1

== system halout/HAL_OUT/CAN4/FD4_CE100_1_0x182/CCUCbnPreEstimdTi ==
  CCUCbnPreEstimdTi : Inport
  Data Type Conversion : DataTypeConversion  OutDataTypeStr=uint8  RndMeth=Round
  CAN4_CCU_CbnPreEstimdTi : Outport
  wires:
  Data Type Conversion/1 -> CAN4_CCU_CbnPreEstimdTi/1
  CCUCbnPreEstimdTi/1 -> Data Type Conversion/1

== system halout/HAL_OUT/CAN4/FD4_CE100_1_0x182/CCUCbnPreSts ==
  CCUCbnPreSts : Inport
  Data Type Conversion : DataTypeConversion  OutDataTypeStr=uint8  RndMeth=Round
  CAN4_CCU_CbnPreSts : Outport
  wires:
  Data Type Conversion/1 -> CAN4_CCU_CbnPreSts/1
  CCUCbnPreSts/1 -> Data Type Conversion/1

== system halout/HAL_OUT/CAN4/FD4_CE100_1_0x182/CCUDispalyRequest ==
  CCUDispalyRequest : Inport
  Data Type Conversion : DataTypeConversion  OutDataTypeStr=uint8  RndMeth=Round
  CAN4_CCU_Dispaly_Request : Outport
  wires:
  Data Type Conversion/1 -> CAN4_CCU_Dispaly_Request/1
  CCUDispalyRequest/1 -> Data Type Conversion/1

== system halout/HAL_OUT/CAN4/FD4_CE100_1_0x182/CCUEcoSts ==
  CCUEcoSts : Inport
  Data Type Conversion : DataTypeConversion  OutDataTypeStr=uint8  RndMeth=Round
  CAN4_CCU_EcoSts : Outport
  wires:
  Data Type Conversion/1 -> CAN4_CCU_EcoSts/1
  CCUEcoSts/1 -> Data Type Conversion/1

== system halout/HAL_OUT/CAN4/FD4_CE100_1_0x182/CCUFrtOnOffLampSts ==
  CCUFrtOnOffLampSts : Inport
  Data Type Conversion : DataTypeConversion  OutDataTypeStr=uint8  RndMeth=Round
  CAN4_CCU_FrtOnOffLampSts : Outport
  wires:
  Data Type Conversion/1 -> CAN4_CCU_FrtOnOffLampSts/1
  CCUFrtOnOffLampSts/1 -> Data Type Conversion/1

== system halout/HAL_OUT/CAN4/FD4_CE100_1_0x182/CCUHEATMaxLampSts ==
  CCUHEATMaxLampSts : Inport
  Data Type Conversion : DataTypeConversion  OutDataTypeStr=uint8  RndMeth=Round
  CAN4_CCU_HEATMaxLampSts : Outport
  wires:
  Data Type Conversion/1 -> CAN4_CCU_HEATMaxLampSts/1
  CCUHEATMaxLampSts/1 -> Data Type Conversion/1

== system halout/HAL_OUT/CAN4/FD4_CE100_1_0x182/CCUHiVoltageReq ==
  CCUHiVoltageReq : Inport
  Data Type Conversion : DataTypeConversion  OutDataTypeStr=uint8  RndMeth=Round
  CAN4_CCU_HiVoltageReq : Outport
  wires:
  Data Type Conversion/1 -> CAN4_CCU_HiVoltageReq/1
  CCUHiVoltageReq/1 -> Data Type Conversion/1

== system halout/HAL_OUT/CAN4/FD4_CE100_1_0x182/CCURrOnOffLampSts ==
  CCURrOnOffLampSts : Inport
  Data Type Conversion : DataTypeConversion  OutDataTypeStr=uint8  RndMeth=Round
  CAN4_CCU_RrOnOffLampSts : Outport
  wires:
  Data Type Conversion/1 -> CAN4_CCU_RrOnOffLampSts/1
  CCURrOnOffLampSts/1 -> Data Type Conversion/1

== system halout/HAL_OUT/CAN4/FD4_CE100_1_0x182/CCUSyncLampSts ==
  CCUSyncLampSts : Inport
  Data Type Conversion : DataTypeConversion  OutDataTypeStr=uint8  RndMeth=Round
  CAN4_CCU_SyncLampSts : Outport
  wires:
  Data Type Conversion/1 -> CAN4_CCU_SyncLampSts/1
  CCUSyncLampSts/1 -> Data Type Conversion/1

== system halout/HAL_OUT/CAN4/FD4_CE100_1_0x182/CabinMode ==
  CabinMode : Inport
  Data Type Conversion : DataTypeConversion  OutDataTypeStr=uint8  RndMeth=Round
  CAN4_CabinMode : Outport
  wires:
  Data Type Conversion/1 -> CAN4_CabinMode/1
  CabinMode/1 -> Data Type Conversion/1

== system halout/HAL_OUT/CAN4/FD4_CE100_1_0x182/CoolgFanActDuty ==
  CoolgFanActDuty : Inport
  Data Type Conversion : DataTypeConversion  OutDataTypeStr=uint8  RndMeth=Round
  convert_out : FVT_lib/hal/convert_out  gain=0.5  offset=0
  CAN4_CoolgFanActDuty : Outport
  wires:
  Data Type Conversion/1 -> CAN4_CoolgFanActDuty/1
  convert_out/1 -> Data Type Conversion/1
  CoolgFanActDuty/1 -> convert_out/1

== system halout/HAL_OUT/CAN4/FD4_CE100_1_0x182/DeiceModReq ==
  DeiceModReq : Inport
  Data Type Conversion : DataTypeConversion  OutDataTypeStr=uint8  RndMeth=Round
  CAN4_DeiceModReq : Outport
  wires:
  Data Type Conversion/1 -> CAN4_DeiceModReq/1
  DeiceModReq/1 -> Data Type Conversion/1

== system halout/HAL_OUT/CAN4/FD4_CE100_1_0x182/EDriveMode ==
  EDriveMode : Inport
  Data Type Conversion : DataTypeConversion  OutDataTypeStr=uint8  RndMeth=Round
  CAN4_EDriveMode : Outport
  wires:
  Data Type Conversion/1 -> CAN4_EDriveMode/1
  EDriveMode/1 -> Data Type Conversion/1

== system halout/HAL_OUT/CAN4/FD4_CE100_1_0x182/FDAGSCmd ==
  FDAGSCmd : Inport
  Data Type Conversion : DataTypeConversion  OutDataTypeStr=uint8  RndMeth=Round
  CAN4_FD_AGS_Cmd : Outport
  wires:
  Data Type Conversion/1 -> CAN4_FD_AGS_Cmd/1
  FDAGSCmd/1 -> Data Type Conversion/1

== system halout/HAL_OUT/CAN4/FD4_CE100_1_0x182/FDBlowerCmd ==
  FDBlowerCmd : Inport
  Data Type Conversion : DataTypeConversion  OutDataTypeStr=uint8  RndMeth=Round
  convert_out : FVT_lib/hal/convert_out  gain=0.8  offset=0
  CAN4_FD_Blower_Cmd : Outport
  wires:
  Data Type Conversion/1 -> CAN4_FD_Blower_Cmd/1
  convert_out/1 -> Data Type Conversion/1
  FDBlowerCmd/1 -> convert_out/1

== system halout/HAL_OUT/CAN4/FD4_CE100_1_0x182/FDCTHCMCLEVentYSta ==
  FDCTHCMCLEVentYSta : Inport
  Data Type Conversion : DataTypeConversion  OutDataTypeStr=uint8  RndMeth=Round
  CAN4_FDC_THCM_CLEVentY_Sta : Outport
  wires:
  Data Type Conversion/1 -> CAN4_FDC_THCM_CLEVentY_Sta/1
  FDCTHCMCLEVentYSta/1 -> Data Type Conversion/1

== system halout/HAL_OUT/CAN4/FD4_CE100_1_0x182/FDCTHCMCLEVentZSta ==
  FDCTHCMCLEVentZSta : Inport
  Data Type Conversion : DataTypeConversion  OutDataTypeStr=uint8  RndMeth=Round
  CAN4_FDC_THCM_CLEVentZ_Sta : Outport
  wires:
  Data Type Conversion/1 -> CAN4_FDC_THCM_CLEVentZ_Sta/1
  FDCTHCMCLEVentZSta/1 -> Data Type Conversion/1

== system halout/HAL_OUT/CAN4/FD4_CE100_1_0x182/FDCTHCMCLVentSta ==
  FDCTHCMCLVentSta : Inport
  Data Type Conversion : DataTypeConversion  OutDataTypeStr=uint8  RndMeth=Round
  CAN4_FDC_THCM_CLVent_Sta : Outport
  wires:
  Data Type Conversion/1 -> CAN4_FDC_THCM_CLVent_Sta/1
  FDCTHCMCLVentSta/1 -> Data Type Conversion/1

== system halout/HAL_OUT/CAN4/FD4_CE100_1_0x182/FDCTHCMCREVentYSta ==
  FDCTHCMCREVentYSta : Inport
  Data Type Conversion : DataTypeConversion  OutDataTypeStr=uint8  RndMeth=Round
  CAN4_FDC_THCM_CREVentY_Sta : Outport
  wires:
  Data Type Conversion/1 -> CAN4_FDC_THCM_CREVentY_Sta/1
  FDCTHCMCREVentYSta/1 -> Data Type Conversion/1

== system halout/HAL_OUT/CAN4/FD4_CE100_1_0x182/FDCTHCMCREVentZSta ==
  FDCTHCMCREVentZSta : Inport
  Data Type Conversion : DataTypeConversion  OutDataTypeStr=uint8  RndMeth=Round
  CAN4_FDC_THCM_CREVentZ_Sta : Outport
  wires:
  Data Type Conversion/1 -> CAN4_FDC_THCM_CREVentZ_Sta/1
  FDCTHCMCREVentZSta/1 -> Data Type Conversion/1

== system halout/HAL_OUT/CAN4/FD4_CE100_1_0x182/FDCTHCMCRVentSta ==
  FDCTHCMCRVentSta : Inport
  Data Type Conversion : DataTypeConversion  OutDataTypeStr=uint8  RndMeth=Round
  CAN4_FDC_THCM_CRVent_Sta : Outport
  wires:
  Data Type Conversion/1 -> CAN4_FDC_THCM_CRVent_Sta/1
  FDCTHCMCRVentSta/1 -> Data Type Conversion/1

== system halout/HAL_OUT/CAN4/FD4_CE100_1_0x182/FDCTHCMLEVentModeSta ==
  FDCTHCMLEVentModeSta : Inport
  Data Type Conversion : DataTypeConversion  OutDataTypeStr=uint8  RndMeth=Round
  CAN4_FDC_THCM_LEVentMode_Sta : Outport
  wires:
  Data Type Conversion/1 -> CAN4_FDC_THCM_LEVentMode_Sta/1
  FDCTHCMLEVentModeSta/1 -> Data Type Conversion/1

== system halout/HAL_OUT/CAN4/FD4_CE100_1_0x182/FDCTHCMLEVentYSta ==
  FDCTHCMLEVentYSta : Inport
  Data Type Conversion : DataTypeConversion  OutDataTypeStr=uint8  RndMeth=Round
  CAN4_FDC_THCM_LEVentY_Sta : Outport
  wires:
  Data Type Conversion/1 -> CAN4_FDC_THCM_LEVentY_Sta/1
  FDCTHCMLEVentYSta/1 -> Data Type Conversion/1

== system halout/HAL_OUT/CAN4/FD4_CE100_1_0x182/FDCTHCMLEVentZSta ==
  FDCTHCMLEVentZSta : Inport
  Data Type Conversion : DataTypeConversion  OutDataTypeStr=uint8  RndMeth=Round
  CAN4_FDC_THCM_LEVentZ_Sta : Outport
  wires:
  Data Type Conversion/1 -> CAN4_FDC_THCM_LEVentZ_Sta/1
  FDCTHCMLEVentZSta/1 -> Data Type Conversion/1

== system halout/HAL_OUT/CAN4/FD4_CE100_1_0x182/FDCTHCMLVentSta ==
  FDCTHCMLVentSta : Inport
  Data Type Conversion : DataTypeConversion  OutDataTypeStr=uint8  RndMeth=Round
  CAN4_FDC_THCM_LVent_Sta : Outport
  wires:
  Data Type Conversion/1 -> CAN4_FDC_THCM_LVent_Sta/1
  FDCTHCMLVentSta/1 -> Data Type Conversion/1

== system halout/HAL_OUT/CAN4/FD4_CE100_1_0x182/FDCTHCMREVentModeSta ==
  FDCTHCMREVentModeSta : Inport
  Data Type Conversion : DataTypeConversion  OutDataTypeStr=uint8  RndMeth=Round
  CAN4_FDC_THCM_REVentMode_Sta : Outport
  wires:
  Data Type Conversion/1 -> CAN4_FDC_THCM_REVentMode_Sta/1
  FDCTHCMREVentModeSta/1 -> Data Type Conversion/1

== system halout/HAL_OUT/CAN4/FD4_CE100_1_0x182/FDCTHCMREVentYSta ==
  FDCTHCMREVentYSta : Inport
  Data Type Conversion : DataTypeConversion  OutDataTypeStr=uint8  RndMeth=Round
  CAN4_FDC_THCM_REVentY_Sta : Outport
  wires:
  Data Type Conversion/1 -> CAN4_FDC_THCM_REVentY_Sta/1
  FDCTHCMREVentYSta/1 -> Data Type Conversion/1

== system halout/HAL_OUT/CAN4/FD4_CE100_1_0x182/FDCTHCMREVentZSta ==
  FDCTHCMREVentZSta : Inport
  Data Type Conversion : DataTypeConversion  OutDataTypeStr=uint8  RndMeth=Round
  CAN4_FDC_THCM_REVentZ_Sta : Outport
  wires:
  Data Type Conversion/1 -> CAN4_FDC_THCM_REVentZ_Sta/1
  FDCTHCMREVentZSta/1 -> Data Type Conversion/1

== system halout/HAL_OUT/CAN4/FD4_CE100_1_0x182/FDCTHCMRVentSta ==
  FDCTHCMRVentSta : Inport
  Data Type Conversion : DataTypeConversion  OutDataTypeStr=uint8  RndMeth=Round
  CAN4_FDC_THCM_RVent_Sta : Outport
  wires:
  Data Type Conversion/1 -> CAN4_FDC_THCM_RVent_Sta/1
  FDCTHCMRVentSta/1 -> Data Type Conversion/1

== system halout/HAL_OUT/CAN4/FD4_CE100_1_0x182/FDCompCmd ==
  FDCompCmd : Inport
  Data Type Conversion : DataTypeConversion  OutDataTypeStr=uint16  RndMeth=Round
  convert_out : FVT_lib/hal/convert_out  gain=0.5  offset=0
  CAN4_FD_Comp_Cmd : Outport
  wires:
  Data Type Conversion/1 -> CAN4_FD_Comp_Cmd/1
  convert_out/1 -> Data Type Conversion/1
  FDCompCmd/1 -> convert_out/1

== system halout/HAL_OUT/CAN4/FD4_CE100_1_0x182/FDEWP1Cmd ==
  FDEWP1Cmd : Inport
  Data Type Conversion : DataTypeConversion  OutDataTypeStr=uint8  RndMeth=Round
  CAN4_FD_EWP1_Cmd : Outport
  wires:
  Data Type Conversion/1 -> CAN4_FD_EWP1_Cmd/1
  FDEWP1Cmd/1 -> Data Type Conversion/1

== system halout/HAL_OUT/CAN4/FD4_CE100_1_0x182/FDEWP2Cmd ==
  FDEWP2Cmd : Inport
  Data Type Conversion : DataTypeConversion  OutDataTypeStr=uint8  RndMeth=Round
  CAN4_FD_EWP2_Cmd : Outport
  wires:
  Data Type Conversion/1 -> CAN4_FD_EWP2_Cmd/1
  FDEWP2Cmd/1 -> Data Type Conversion/1

== system halout/HAL_OUT/CAN4/FD4_CE100_1_0x182/FDEWP3Cmd ==
  FDEWP3Cmd : Inport
  Data Type Conversion : DataTypeConversion  OutDataTypeStr=uint8  RndMeth=Round
  CAN4_FD_EWP3_Cmd : Outport
  wires:
  Data Type Conversion/1 -> CAN4_FD_EWP3_Cmd/1
  FDEWP3Cmd/1 -> Data Type Conversion/1

== system halout/HAL_OUT/CAN4/FD4_CE100_1_0x182/FDEXV1Cmd ==
  FDEXV1Cmd : Inport
  Data Type Conversion : DataTypeConversion  OutDataTypeStr=uint16  RndMeth=Round
  CAN4_FD_EXV1_Cmd : Outport
  wires:
  Data Type Conversion/1 -> CAN4_FD_EXV1_Cmd/1
  FDEXV1Cmd/1 -> Data Type Conversion/1

== system halout/HAL_OUT/CAN4/FD4_CE100_1_0x182/FDEXV2Cmd ==
  FDEXV2Cmd : Inport
  Data Type Conversion : DataTypeConversion  OutDataTypeStr=uint16  RndMeth=Round
  CAN4_FD_EXV2_Cmd : Outport
  wires:
  Data Type Conversion/1 -> CAN4_FD_EXV2_Cmd/1
  FDEXV2Cmd/1 -> Data Type Conversion/1

== system halout/HAL_OUT/CAN4/FD4_CE100_1_0x182/FDFWVCmd ==
  FDFWVCmd : Inport
  Data Type Conversion : DataTypeConversion  OutDataTypeStr=uint8  RndMeth=Round
  CAN4_FD_FWV_Cmd : Outport
  wires:
  Data Type Conversion/1 -> CAN4_FD_FWV_Cmd/1
  FDFWVCmd/1 -> Data Type Conversion/1

== system halout/HAL_OUT/CAN4/FD4_CE100_1_0x182/FDFrLeAPTCHeatPwrCmd ==
  FDFrLeAPTCHeatPwrCmd : Inport
  Data Type Conversion : DataTypeConversion  OutDataTypeStr=uint8  RndMeth=Round
  convert_out : FVT_lib/hal/convert_out  gain=25  offset=0
  CAN4_FD_FrLeAPTCHeatPwr_Cmd : Outport
  wires:
  Data Type Conversion/1 -> CAN4_FD_FrLeAPTCHeatPwr_Cmd/1
  convert_out/1 -> Data Type Conversion/1
  FDFrLeAPTCHeatPwrCmd/1 -> convert_out/1

== system halout/HAL_OUT/CAN4/FD4_CE100_1_0x182/FDFrRiAPTCHeatPwrCmd ==
  FDFrRiAPTCHeatPwrCmd : Inport
  Data Type Conversion : DataTypeConversion  OutDataTypeStr=uint8  RndMeth=Round
  convert_out : FVT_lib/hal/convert_out  gain=25  offset=0
  CAN4_FD_FrRiAPTCHeatPwr_Cmd : Outport
  wires:
  Data Type Conversion/1 -> CAN4_FD_FrRiAPTCHeatPwr_Cmd/1
  convert_out/1 -> Data Type Conversion/1
  FDFrRiAPTCHeatPwrCmd/1 -> convert_out/1

== system halout/HAL_OUT/CAN4/FD4_CE100_1_0x182/FDFrWPTCHeatPwrCmd ==
  FDFrWPTCHeatPwrCmd : Inport
  Data Type Conversion : DataTypeConversion  OutDataTypeStr=uint16  RndMeth=Round
  CAN4_FD_FrWPTCHeatPwr_Cmd : Outport
  wires:
  Data Type Conversion/1 -> CAN4_FD_FrWPTCHeatPwr_Cmd/1
  FDFrWPTCHeatPwrCmd/1 -> Data Type Conversion/1

== system halout/HAL_OUT/CAN4/FD4_CE100_1_0x182/FDRecyAutoCmd ==
  FDRecyAutoCmd : Inport
  Data Type Conversion : DataTypeConversion  OutDataTypeStr=uint8  RndMeth=Round
  CAN4_FD_RecyAuto_Cmd : Outport
  wires:
  Data Type Conversion/1 -> CAN4_FD_RecyAuto_Cmd/1
  FDRecyAutoCmd/1 -> Data Type Conversion/1

== system halout/HAL_OUT/CAN4/FD4_CE100_1_0x182/FDRrAPTCHeatPwrCmd ==
  FDRrAPTCHeatPwrCmd : Inport
  Data Type Conversion : DataTypeConversion  OutDataTypeStr=uint8  RndMeth=Round
  convert_out : FVT_lib/hal/convert_out  gain=25  offset=0
  CAN4_FD_RrAPTCHeatPwr_Cmd : Outport
  wires:
  Data Type Conversion/1 -> CAN4_FD_RrAPTCHeatPwr_Cmd/1
  convert_out/1 -> Data Type Conversion/1
  FDRrAPTCHeatPwrCmd/1 -> convert_out/1

== system halout/HAL_OUT/CAN4/FD4_CE100_1_0x182/FDSOTXVCmd ==
  FDSOTXVCmd : Inport
  Data Type Conversion : DataTypeConversion  OutDataTypeStr=uint8  RndMeth=Round
  CAN4_FD_SOTXV_Cmd : Outport
  wires:
  Data Type Conversion/1 -> CAN4_FD_SOTXV_Cmd/1
  FDSOTXVCmd/1 -> Data Type Conversion/1

== system halout/HAL_OUT/CAN4/FD4_CE100_1_0x182/FDSOV1Cmd ==
  FDSOV1Cmd : Inport
  Data Type Conversion : DataTypeConversion  OutDataTypeStr=uint8  RndMeth=Round
  CAN4_FD_SOV1_Cmd : Outport
  wires:
  Data Type Conversion/1 -> CAN4_FD_SOV1_Cmd/1
  FDSOV1Cmd/1 -> Data Type Conversion/1

== system halout/HAL_OUT/CAN4/FD4_CE100_1_0x182/FDSOV2Cmd ==
  FDSOV2Cmd : Inport
  Data Type Conversion : DataTypeConversion  OutDataTypeStr=uint8  RndMeth=Round
  CAN4_FD_SOV2_Cmd : Outport
  wires:
  Data Type Conversion/1 -> CAN4_FD_SOV2_Cmd/1
  FDSOV2Cmd/1 -> Data Type Conversion/1

== system halout/HAL_OUT/CAN4/FD4_CE100_1_0x182/FDSOV3Cmd ==
  FDSOV3Cmd : Inport
  Data Type Conversion : DataTypeConversion  OutDataTypeStr=uint8  RndMeth=Round
  CAN4_FD_SOV3_Cmd : Outport
  wires:
  Data Type Conversion/1 -> CAN4_FD_SOV3_Cmd/1
  FDSOV3Cmd/1 -> Data Type Conversion/1

== system halout/HAL_OUT/CAN4/FD4_CE100_1_0x182/FDTWVCmd ==
  FDTWVCmd : Inport
  Data Type Conversion : DataTypeConversion  OutDataTypeStr=uint8  RndMeth=Round
  convert_out : FVT_lib/hal/convert_out  gain=0.392  offset=0
  CAN4_FD_TWV_Cmd : Outport
  wires:
  Data Type Conversion/1 -> CAN4_FD_TWV_Cmd/1
  convert_out/1 -> Data Type Conversion/1
  FDTWVCmd/1 -> convert_out/1

== system halout/HAL_OUT/CAN4/FD4_CE100_1_0x182/FrCoolantflow ==
  FrCoolantflow : Inport
  Data Type Conversion : DataTypeConversion  OutDataTypeStr=uint8  RndMeth=Round
  convert_out : FVT_lib/hal/convert_out  gain=0.25  offset=0
  CAN4_Fr_Coolantflow : Outport
  wires:
  Data Type Conversion/1 -> CAN4_Fr_Coolantflow/1
  convert_out/1 -> Data Type Conversion/1
  FrCoolantflow/1 -> convert_out/1

== system halout/HAL_OUT/CAN4/FD4_CE100_1_0x182/FrCoolanttemp ==
  FrCoolanttemp : Inport
  Data Type Conversion : DataTypeConversion  OutDataTypeStr=uint16  RndMeth=Round
  convert_out : FVT_lib/hal/convert_out  gain=1  offset=-40
  CAN4_Fr_Coolanttemp : Outport
  wires:
  Data Type Conversion/1 -> CAN4_Fr_Coolanttemp/1
  convert_out/1 -> Data Type Conversion/1
  FrCoolanttemp/1 -> convert_out/1

== system halout/HAL_OUT/CAN4/FD4_CE100_1_0x182/HPThermalRecoveryReq ==
  HPThermalRecoveryReq : Inport
  Data Type Conversion : DataTypeConversion  OutDataTypeStr=uint8  RndMeth=Round
  CAN4_HPThermalRecoveryReq : Outport
  wires:
  Data Type Conversion/1 -> CAN4_HPThermalRecoveryReq/1
  HPThermalRecoveryReq/1 -> Data Type Conversion/1

== system halout/HAL_OUT/CAN4/FD4_CE100_1_0x182/RrCoolantflow ==
  RrCoolantflow : Inport
  Data Type Conversion : DataTypeConversion  OutDataTypeStr=uint8  RndMeth=Round
  convert_out : FVT_lib/hal/convert_out  gain=0.25  offset=0
  CAN4_Rr_Coolantflow : Outport
  wires:
  Data Type Conversion/1 -> CAN4_Rr_Coolantflow/1
  convert_out/1 -> Data Type Conversion/1
  RrCoolantflow/1 -> convert_out/1
